simulink model "model"  (R2022b)
settings: Solver=VariableStepAuto  StartTime=0.0  StopTime=100  RelTol=1e-3
model workspace (MAT data in the model file):
  a1 = 1
  kp = 15
  kt = 20
  m = 30
  u = 10
settings Model: Creator=markm  LastModifiedBy=markm

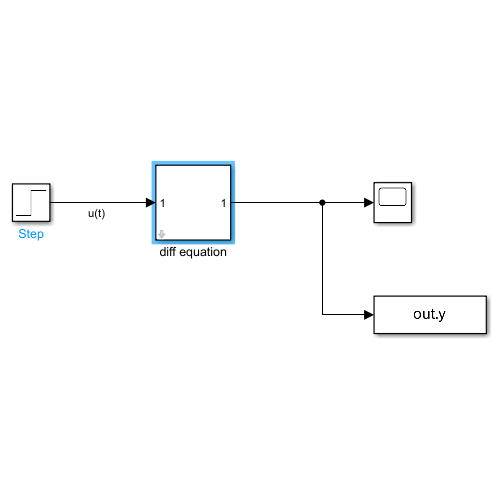
[thumbnail: Simulink's stored preview of the top-level diagram]
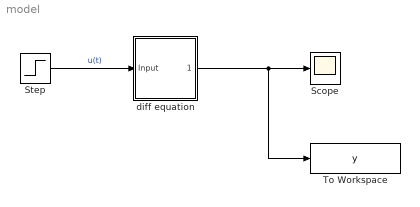
== system model ==
  Scope : Scope
  Step : Step  After=10  SampleTime=0
  To Workspace : ToWorkspace  VariableName=y  SaveFormat=Timeseries  SampleTime=-1
  diff equation : Subsystem  mask{kp=15, kt=20, m=30}
  wires:
  diff equation/1(Output) -> To Workspace/1, Scope/1
  Step/1 -> diff equation/1(Input)  "u(t)"

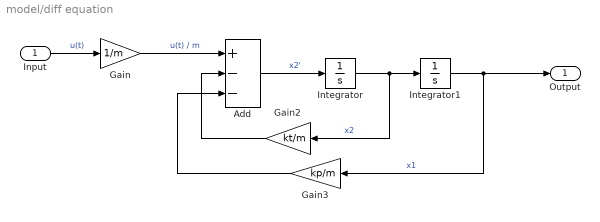
== system model/diff equation ==
  Input : Inport
  Add : Sum  Inputs=+--
  Gain : Gain  Gain=1/m
  Gain2 : Gain  Gain=kt/m
  Gain3 : Gain  Gain=kp/m
  Integrator : Integrator
  Integrator1 : Integrator
  Output : Outport
  wires:
  Add/1 -> Integrator/1  "x2'"
  Integrator/1 -> Gain2/1, Integrator1/1  "x2"
  Input/1 -> Gain/1  "u(t)"
  Integrator1/1 -> Output/1, Gain3/1  "x1"
  Gain3/1 -> Add/3
  Gain2/1 -> Add/2
  Gain/1 -> Add/1  "u(t) / m"
